simulink model "QRsim"  (R2013b)
settings: Solver=ode45  StartTime=0.0  StopTime=15  RelTol=1e-3
values from neighbouring files (symbols this model uses):
  b = 1    [QRrunfile.m]    (also in develop.m = 0.1)
  d = 8.004e-4    (= 0.0008004)    [QRrunfile.m]    (also in develop.m = 0.1)
  DeltaR = [0; 0; 0]    [QRrunfile.m]
  Deltax = [0; 0; 0]    [QRrunfile.m]
  dphi0 = 0    [QRrunfile.m]    (also in develop.m)
  dpsi0 = 0    [QRrunfile.m]    (also in develop.m)
  dtheta0 = 0    [QRrunfile.m]    (also in develop.m)
  dx0 = 0    [QRrunfile.m]    (also in develop.m)
  dy0 = 0    [QRrunfile.m]    (also in develop.m)
  dz0 = 0    [QRrunfile.m]    (also in develop.m)
  e3 = [0;0;1]    [QRrunfile.m]
  g = 9.81    [QRrunfile.m]    (also in develop.m)
  I = diag([Ixx Iyy Izz])    [QRrunfile.m]    (also in develop.m)
  Ir = 0    [QRrunfile.m]    (also in develop.m = 0.5)
  Ixx = 0.0820    (= 0.082)    [QRrunfile.m]    (also in develop.m = 1.5)
  Iyy = 0.0845    [QRrunfile.m]    (also in develop.m = 1.5)
  Izz = .1377    (= 0.1377)    [QRrunfile.m]    (also in develop.m = 1.5)
  kOmega = kOmega_phi*eye(3)    [QRrunfile.m]
  kR = kR_phi*eye(3)    [QRrunfile.m]
  kv = 5.6*m    (= 24.304)    [QRrunfile.m]
  kx = 16*m    (= 69.44)    [QRrunfile.m]
  l = 0.315    [QRrunfile.m]    (also in develop.m = 0.12)
  m = 4.34    [QRrunfile.m]    (also in develop.m = 0.42)
  phi0 = pi/8    (= 0.392699081699)    [QRrunfile.m]    (also in develop.m = 0)
  psi0 = 0    [QRrunfile.m]    (also in develop.m)
  theta0 = 0    [QRrunfile.m]    (also in develop.m)
  x0 = 0    [QRrunfile.m]    (also in develop.m)
  y0 = 0    [QRrunfile.m]    (also in develop.m)
  z0 = 0    [QRrunfile.m]    (also in develop.m)
undefined symbols (not defined in the file or in its folder): sigbuilder_block
libraries: dspsrcs4 x3, simulink_extras x3, vrlib x1
settings Model: Creator=Nam  LastModifiedBy=Nam
settings DataIOCC: SaveFormat=StructureWithTime
settings DebuggingCC: SolverPrmCheckMsg=none

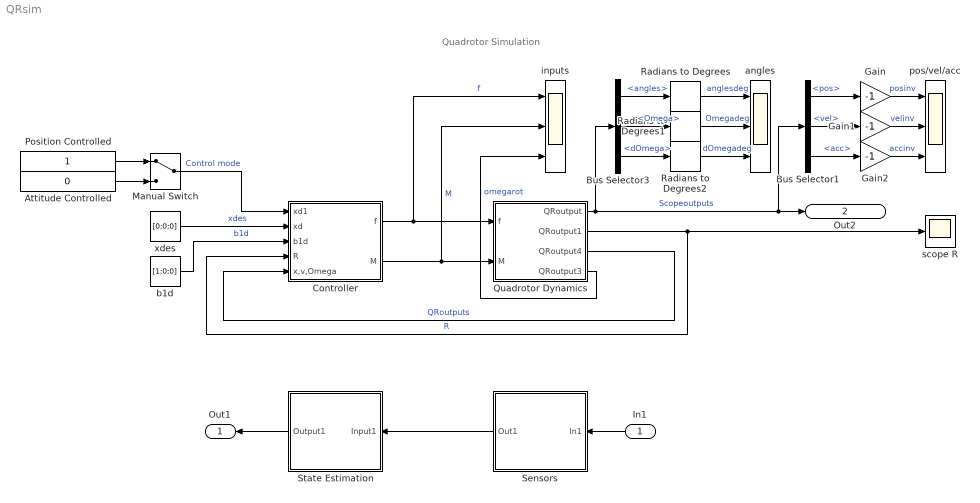
== system QRsim ==
  note: Quadrotor Simulation
  In1 : Inport
  Attitude Controlled : Constant  Value=0  VectorParams1D=off
      mask Display: disp('Attitude controlled')
  Bus Selector1 : BusSelector  OutputSignals=signal1.pos,signal1.vel,signal1.acc
  Bus Selector3 : BusSelector  OutputSignals=signal2.angles,signal2.Omega,signal2.dOmega
  Controller : Subsystem
      mask Display: disp('Controller')
  Gain : Gain  Gain=-1
  Gain1 : Gain  Gain=-1
  Gain2 : Gain  Gain=-1
  Manual Switch : ManualSwitch
  Position Controlled : Constant  VectorParams1D=off
      mask Display: disp('Position controlled')
  Quadrotor Dynamics : Subsystem
      mask Display: image('bebop.png')
  Radians to Degrees : simulink_extras/Transformations/Radians to Degrees
  Radians to Degrees1 : simulink_extras/Transformations/Radians to Degrees
  Radians to Degrees2 : simulink_extras/Transformations/Radians to Degrees
  Sensors : Subsystem
      mask Display: image('optitrack.jpg')
  State Estimation : Subsystem
  angles : Scope  NumInputPorts=3
      settings: ShowLegends=on  YMin=-375~-850~-1e+13  YMax=25~0~1e+12
  b1d : Constant  Value=[1;0;0]  VectorParams1D=off
  inputs : Scope  NumInputPorts=3
      settings: ShowLegends=on  YMin=-5~-5~-5  YMax=5~5~5  SaveName=ScopeData2
  pos/vel/acc : Scope  NumInputPorts=3
      settings: ShowLegends=on  YMin=-5~-5~-5  YMax=5~5~5
  scope R : Scope
      settings: SaveName=ScopeData16
  xdes : Constant  Value=[0;0;0]  VectorParams1D=off
  Out1 : Outport
  Out2 : Outport  Port=2
  wires:
  Sensors/1(Out1) -> State Estimation/1(Input1)
  xdes/1 -> Controller/2(xd)  "xdes"
  b1d/1 -> Controller/3(b1d)  "b1d"
  State Estimation/1(Output1) -> Out1/1
  In1/1 -> Sensors/1(In1)
  Controller/1(f) -> Quadrotor Dynamics/1(f), inputs/1  "f"
  Controller/2(M) -> Quadrotor Dynamics/2(M), inputs/2  "M"
  Quadrotor Dynamics/1(QRoutput) -> Bus Selector1/1, Out2/1, Bus Selector3/1  "Scopeoutputs"
  Bus Selector3/1 -> Radians to Degrees/1  "<angles>"
  Bus Selector3/2 -> Radians to Degrees1/1  "<Omega>"
  Bus Selector3/3 -> Radians to Degrees2/1  "<dOmega>"
  Gain/1 -> pos/vel/acc/1  "posinv"
  Gain1/1 -> pos/vel/acc/2  "velinv"
  Gain2/1 -> pos/vel/acc/3  "accinv"
  Bus Selector1/1 -> Gain/1  "<pos>"
  Bus Selector1/2 -> Gain1/1  "<vel>"
  Bus Selector1/3 -> Gain2/1  "<acc>"
  Quadrotor Dynamics/4(QRoutput3) -> inputs/3  "omegarot"
  Quadrotor Dynamics/2(QRoutput1) -> scope R/1, Controller/4(R)  "R"
  Quadrotor Dynamics/3(QRoutput4) -> Controller/5(x,v,Omega)  "QRoutputs"
  Radians to Degrees/1 -> angles/1  "anglesdeg"
  Radians to Degrees1/1 -> angles/2  "Omegadeg"
  Radians to Degrees2/1 -> angles/3  "dOmegadeg"
  Position Controlled/1 -> Manual Switch/1
  Attitude Controlled/1 -> Manual Switch/2
  Manual Switch/1 -> Controller/1(xd1)  "Control mode"

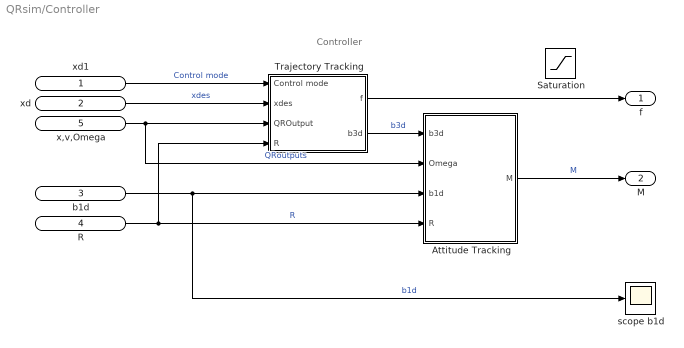
== system QRsim/Controller ==
  note: Controller
  xd1 : Inport
  xd : Inport  Port=2
  b1d : Inport  Port=3
  R : Inport  Port=4
  x,v,Omega : Inport  Port=5
  Attitude Tracking : Subsystem
      mask Display: disp('Attitude\nTracking')
  Saturation : Saturate  UpperLimit=200  LowerLimit=-200
  Trajectory Tracking : Subsystem
      mask Display: disp('Trajectory\nTracking')
  scope b1d : Scope
      settings: SaveName=ScopeData5
  f : Outport
  M : Outport  Port=2
  wires:
  b1d/1 -> scope b1d/1, Attitude Tracking/3(b1d)  "b1d"
  Attitude Tracking/1(M) -> M/1  "M"
  xd/1 -> Trajectory Tracking/2(xdes)  "xdes"
  Trajectory Tracking/2(b3d) -> Attitude Tracking/1(b3d)  "b3d"
  R/1 -> Trajectory Tracking/4(R), Attitude Tracking/4(R)  "R"
  x,v,Omega/1 -> Attitude Tracking/2(Omega), Trajectory Tracking/3(QROutput)  "QRoutputs"
  Trajectory Tracking/1(f) -> f/1
  xd1/1 -> Trajectory Tracking/1(Control mode)  "Control mode"

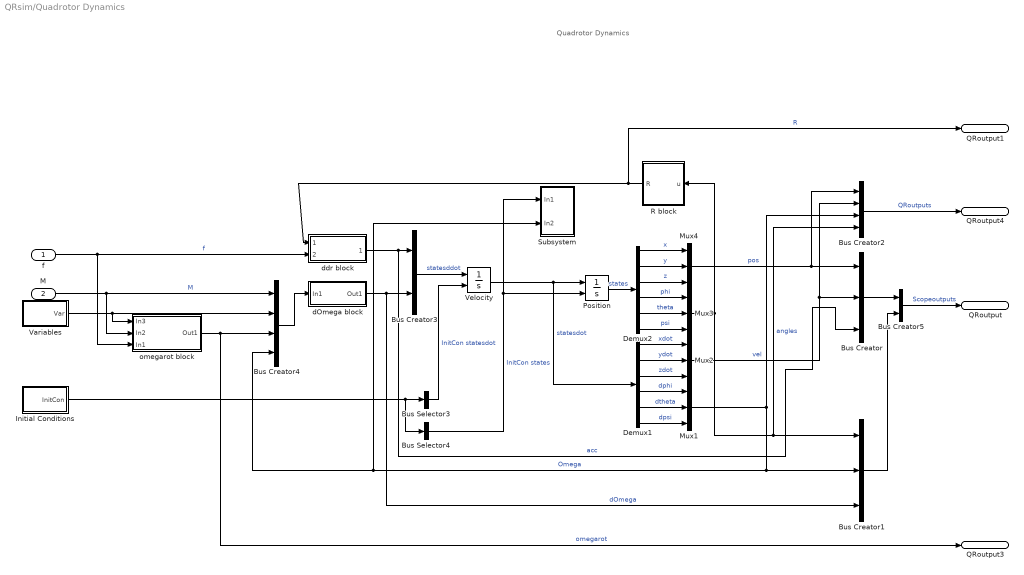
== system QRsim/Quadrotor Dynamics ==
  note: Quadrotor Dynamics
  f : Inport
  M : Inport  Port=2  PortDimensions=[3 1]
  Bus Creator : BusCreator  Inputs=3
  Bus Creator1 : BusCreator  Inputs=3
  Bus Creator2 : BusCreator
  Bus Creator3 : BusCreator  Inputs=2
  Bus Creator4 : BusCreator
  Bus Creator5 : BusCreator  Inputs=2
  Bus Selector3 : BusSelector  OutputSignals=InitCon dot.dx0,InitCon dot.dy0,InitCon dot.dz0,InitCon dot.dphi0,InitCon dot.dtheta0,InitCon dot.dpsi0  OutputAsBus=on
  Bus Selector4 : BusSelector  OutputSignals=InitCon.x0,InitCon.y0,InitCon.z0,InitCon.phi0,InitCon.theta0,InitCon.psi0  OutputAsBus=on
  Demux1 : Demux  Outputs=6
  Demux2 : Demux  Outputs=6
  Initial Conditions : Subsystem
  Mux{1..4} (4 alike) : Mux  Inputs=3
  Position : Integrator  InitialConditionSource=external
  R block : MATLAB Function  TreatAsAtomicUnit=on
  Subsystem : Subsystem
  Variables : Subsystem
      mask Display: disp('Variables')
  Velocity : Integrator  InitialConditionSource=external
  dOmega block : Subsystem
      mask Display: disp('[\psi{"}; \phi{"}; \theta{"}]','texmode','on')
  ddr block : Subsystem
      mask Display: disp('[x{"}; y{"}; z{"}]','texmode','on')
  omegarot block : Subsystem
      mask Display: disp('(f,M) \rightarrow \omega_i','texmode','on')
  QRoutput : Outport
  QRoutput1 : Outport  Port=2
  QRoutput4 : Outport  Port=3
  QRoutput3 : Outport  Port=4
  wires:
  Velocity/1 -> Position/1, Demux1/1  "statesdot"
  f/1 -> ddr block/2(R,f,m,g), omegarot block/3(In1)  "f"
  Variables/1(Var) -> omegarot block/1(In3), Bus Creator4/2
  M/1 -> omegarot block/2(In2), Bus Creator4/1  "M"
  Position/1 -> Demux2/1  "states"
  ddr block/1(rddotOutput) -> Bus Creator/3, Bus Creator3/1  "acc"
  Bus Creator3/1 -> Velocity/1  "statesddot"
  Initial Conditions/1(InitCon) -> Bus Selector3/1, Bus Selector4/1
  Bus Selector3/1 -> Velocity/2  "InitCon statesdot"
  Bus Selector4/1 -> Subsystem/1(In1), Position/2  "InitCon states"
  dOmega block/1(Out1) -> Bus Creator3/2, Bus Creator1/3  "dOmega"
  Bus Creator4/1 -> dOmega block/1(In1)
  Demux1/4 -> Mux1/1  "dphi"
  Demux1/5 -> Mux1/2  "dtheta"
  Demux1/6 -> Mux1/3  "dpsi"
  Demux1/2 -> Mux2/2  "ydot"
  Demux1/1 -> Mux2/1  "xdot"
  Demux1/3 -> Mux2/3  "zdot"
  Mux2/1 -> Bus Creator2/2, Bus Creator/2  "vel"
  Demux2/4 -> Mux3/1  "phi"
  Demux2/5 -> Mux3/2  "theta"
  Demux2/6 -> Mux3/3  "psi"
  Demux2/2 -> Mux4/2  "y"
  Demux2/1 -> Mux4/1  "x"
  Demux2/3 -> Mux4/3  "z"
  Mux3/1 -> Bus Creator2/4, Bus Creator1/1, R block/1(u)  "angles"
  Mux4/1 -> Bus Creator2/1, Bus Creator/1  "pos"
  omegarot block/1(Out1) -> QRoutput3/1, Bus Creator4/3  "omegarot"
  Bus Creator/1 -> Bus Creator5/1
  Bus Creator1/1 -> Bus Creator5/2
  Bus Creator5/1 -> QRoutput/1  "Scopeoutputs"
  Mux1/1 -> Subsystem/2(In2), Bus Creator4/4, Bus Creator1/2, Bus Creator2/3  "Omega"
  Bus Creator2/1 -> QRoutput4/1  "QRoutputs"
  R block/1(R) -> QRoutput1/1, ddr block/1(R,f,m,g1)  "R"

== system QRsim/Sensors ==
  In1 : Inport
  Out1 : Outport
  wires:
  In1/1 -> Out1/1

== system QRsim/State Estimation ==
  Input1 : Inport
  Output1 : Outport
  wires:
  Input1/1 -> Output1/1

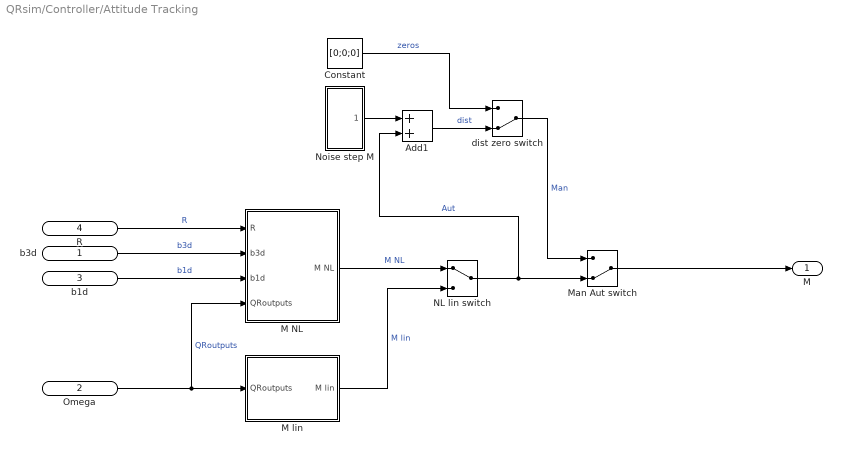
== system QRsim/Controller/Attitude Tracking ==
  b3d : Inport
  Omega : Inport  Port=2
  b1d : Inport  Port=3
  R : Inport  Port=4
  Add1 : Sum
  Constant : Constant  Value=[0;0;0]
  M NL : Subsystem
  M lin : Subsystem
  Man Aut switch : ManualSwitch  CurrentSetting=0
  NL lin switch : ManualSwitch
  Noise step M : Subsystem
  dist zero switch : ManualSwitch  CurrentSetting=0
  M : Outport
  wires:
  M NL/1(M NL) -> NL lin switch/1  "M NL"
  R/1 -> M NL/1(R)  "R"
  b3d/1 -> M NL/2(b3d)  "b3d"
  b1d/1 -> M NL/3(b1d)  "b1d"
  Omega/1 -> M NL/4(QRoutputs), M lin/1(QRoutputs)  "QRoutputs"
  M lin/1(M lin) -> NL lin switch/2  "M lin"
  Noise step M/1(Out1) -> Add1/1
  Constant/1 -> dist zero switch/1  "zeros"
  Add1/1 -> dist zero switch/2  "dist"
  dist zero switch/1 -> Man Aut switch/1  "Man"
  NL lin switch/1 -> Add1/2, Man Aut switch/2  "Aut"
  Man Aut switch/1 -> M/1

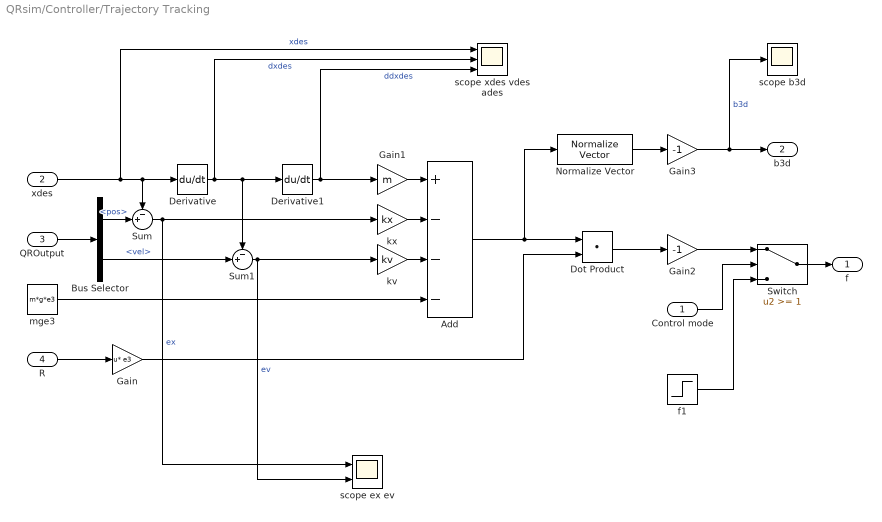
== system QRsim/Controller/Trajectory Tracking ==
  Control mode : Inport
  xdes : Inport  Port=2
  QROutput : Inport  Port=3
  R : Inport  Port=4
  Add : Sum  Inputs=+---
  Bus Selector : BusSelector  OutputSignals=pos,vel
  Derivative : Derivative
  Derivative1 : Derivative
  Dot Product : DotProduct  InputSameDT=on  OutDataTypeStr=Inherit: Inherit via internal rule
  Gain : Gain  Gain=e3  Multiplication=Matrix(u*K)
  Gain1 : Gain  Gain=m
  Gain2 : Gain  Gain=-1
  Gain3 : Gain  Gain=-1
  Normalize Vector : vrlib/Utilities/Normalize Vector  maxzero=0
  Sum : Sum  Inputs=-+|
  Sum1 : Sum  Inputs=-+|
  Switch : Switch  Threshold=1
  f1 : Step  Time=0  After=m*g  SampleTime=0
  kv : Gain  Gain=kv
  kx : Gain  Gain=kx
  mge3 : Constant  Value=m*g*e3  VectorParams1D=off
  scope b3d : Scope
      settings: SaveName=ScopeData4
  scope ex ev : Scope  NumInputPorts=2
      settings: YMin=-5~-5  YMax=5~5  SaveName=ScopeData7
  scope xdes vdes ades : Scope  NumInputPorts=3
      settings: YMin=-5~-5~-5  YMax=5~5~5  SaveName=ScopeData6
  f : Outport
  b3d : Outport  Port=2
  wires:
  xdes/1 -> Derivative/1, Sum/1, scope xdes vdes ades/1  "xdes"
  Derivative/1 -> Derivative1/1, Sum1/1, scope xdes vdes ades/2  "dxdes"
  Derivative1/1 -> Gain1/1, scope xdes vdes ades/3  "ddxdes"
  QROutput/1 -> Bus Selector/1
  Bus Selector/1 -> Sum/2  "<pos>"
  Bus Selector/2 -> Sum1/2  "<vel>"
  R/1 -> Gain/1
  Sum1/1 -> scope ex ev/2, kv/1  "ev"
  Sum/1 -> scope ex ev/1, kx/1  "ex"
  Gain1/1 -> Add/1
  kx/1 -> Add/2
  kv/1 -> Add/3
  mge3/1 -> Add/4
  Dot Product/1 -> Gain2/1
  Add/1 -> Normalize Vector/1, Dot Product/1
  Gain/1 -> Dot Product/2
  Normalize Vector/1 -> Gain3/1
  Gain3/1 -> scope b3d/1, b3d/1  "b3d"
  Gain2/1 -> Switch/1
  f1/1 -> Switch/3
  Switch/1 -> f/1
  Control mode/1 -> Switch/2

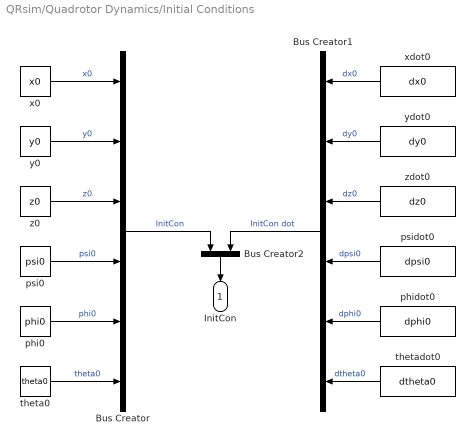
== system QRsim/Quadrotor Dynamics/Initial Conditions ==
  Bus Creator : BusCreator  Inputs=6
  Bus Creator1 : BusCreator  Inputs=6
  Bus Creator2 : BusCreator  Inputs=2
  phi0 : Constant  Value=phi0
  phidot0 : Constant  Value=dphi0
  psi0 : Constant  Value=psi0
  psidot0 : Constant  Value=dpsi0
  theta0 : Constant  Value=theta0
  thetadot0 : Constant  Value=dtheta0
  x0 : Constant  Value=x0
  xdot0 : Constant  Value=dx0
  y0 : Constant  Value=y0
  ydot0 : Constant  Value=dy0
  z0 : Constant  Value=z0
  zdot0 : Constant  Value=dz0
  InitCon : Outport
  wires:
  phi0/1 -> Bus Creator/5  "phi0"
  y0/1 -> Bus Creator/2  "y0"
  psi0/1 -> Bus Creator/4  "psi0"
  x0/1 -> Bus Creator/1  "x0"
  z0/1 -> Bus Creator/3  "z0"
  theta0/1 -> Bus Creator/6  "theta0"
  Bus Creator1/1 -> Bus Creator2/2  "InitCon dot"
  psidot0/1 -> Bus Creator1/4  "dpsi0"
  xdot0/1 -> Bus Creator1/1  "dx0"
  zdot0/1 -> Bus Creator1/3  "dz0"
  ydot0/1 -> Bus Creator1/2  "dy0"
  phidot0/1 -> Bus Creator1/5  "dphi0"
  thetadot0/1 -> Bus Creator1/6  "dtheta0"
  Bus Creator2/1 -> InitCon/1
  Bus Creator/1 -> Bus Creator2/1  "InitCon"

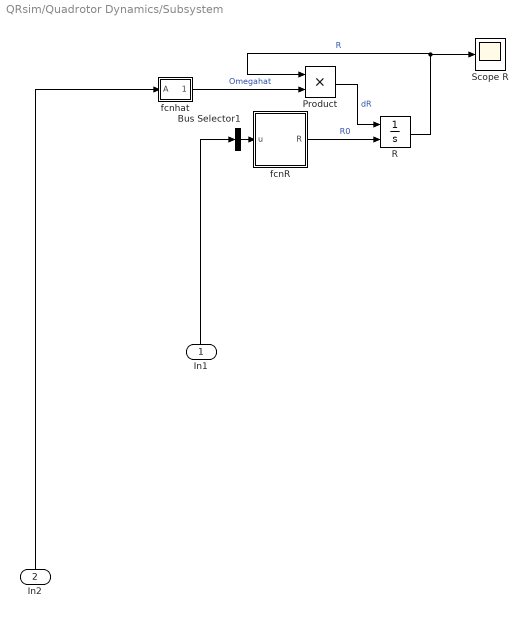
== system QRsim/Quadrotor Dynamics/Subsystem ==
  In1 : Inport
  In2 : Inport  Port=2
  Bus Selector1 : BusSelector  OutputSignals=phi0,theta0,psi0  OutputAsBus=on
  Product : Product
  R : Integrator  InitialConditionSource=external
  Scope R : Scope
      settings: ShowLegends=on  SaveName=ScopeData9
  fcnR : MATLAB Function  TreatAsAtomicUnit=on
  fcnhat : MATLAB Function  TreatAsAtomicUnit=on
  wires:
  Bus Selector1/1 -> fcnR/1(u)
  In2/1 -> fcnhat/1(A)
  In1/1 -> Bus Selector1/1
  fcnhat/1(fcnhat) -> Product/2  "Omegahat"
  fcnR/1(R) -> R/2  "R0"
  Product/1 -> R/1  "dR"
  R/1 -> Scope R/1, Product/1  "R"

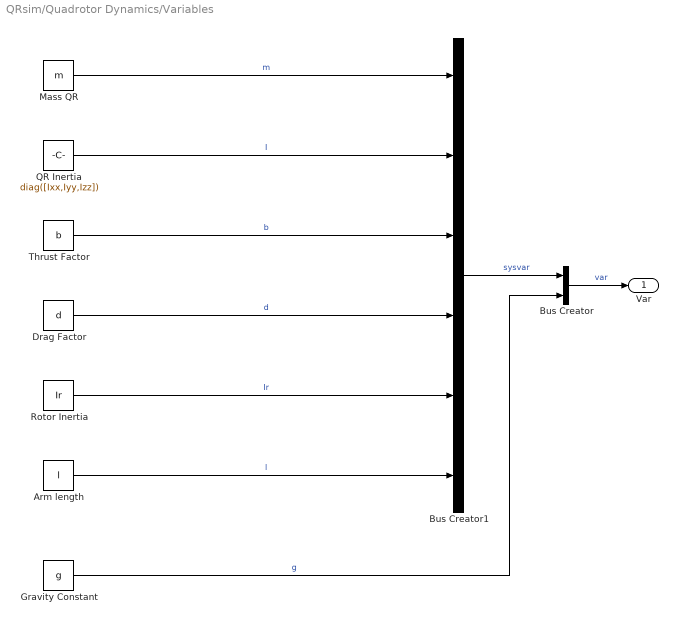
== system QRsim/Quadrotor Dynamics/Variables ==
  Arm length : Constant  Value=l
  Bus Creator : BusCreator  Inputs=2
  Bus Creator1 : BusCreator  Inputs=6
  Drag Factor : Constant  Value=d
  Gravity Constant : Constant  Value=g
  Mass QR : Constant  Value=m
  QR Inertia : Constant  Value=diag([Ixx,Iyy,Izz])
  Rotor Inertia : Constant  Value=Ir
  Thrust Factor : Constant  Value=b
  Var : Outport
  wires:
  Gravity Constant/1 -> Bus Creator/2  "g"
  Bus Creator/1 -> Var/1  "var"
  Mass QR/1 -> Bus Creator1/1  "m"
  Arm length/1 -> Bus Creator1/6  "l"
  Rotor Inertia/1 -> Bus Creator1/5  "Ir"
  QR Inertia/1 -> Bus Creator1/2  "I"
  Bus Creator1/1 -> Bus Creator/1  "sysvar"
  Thrust Factor/1 -> Bus Creator1/3  "b"
  Drag Factor/1 -> Bus Creator1/4  "d"

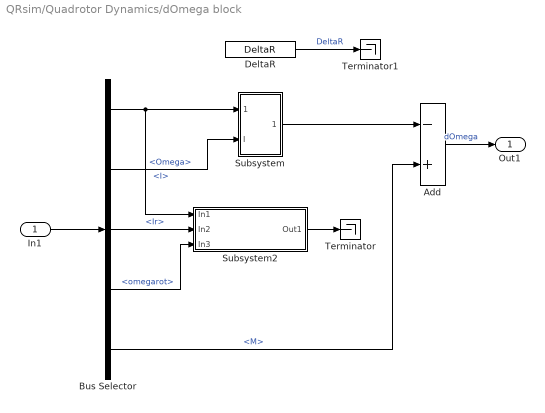
== system QRsim/Quadrotor Dynamics/dOmega block ==
  In1 : Inport
  Add : Sum  Inputs=-+
  Bus Selector : BusSelector  OutputSignals=Omega,var.sysvar.I,var.sysvar.Ir,omegarot,M
  DeltaR : Constant  Value=DeltaR
      mask Display: disp('\Delta_R','texmode','on')
  Subsystem : Subsystem
      mask Display: disp('\Omega \times I\Omega','texmode','on')
  Subsystem2 : Subsystem
      mask Display: disp('\tau_G=\Sigma I_R(\omega \times e_3) \omega_i ','texmode','on')
  Terminator : Terminator
  Terminator1 : Terminator
  Out1 : Outport
  wires:
  In1/1 -> Bus Selector/1
  Add/1 -> Out1/1  "dOmega"
  Bus Selector/1 -> Subsystem/1(Omega), Subsystem2/1(In1)  "<Omega>"
  Bus Selector/2 -> Subsystem/2(I)  "<I>"
  Subsystem/1(Out1) -> Add/1
  Bus Selector/3 -> Subsystem2/2(In2)  "<Ir>"
  Bus Selector/5 -> Add/2  "<M>"
  Subsystem2/1(Out1) -> Terminator/1
  Bus Selector/4 -> Subsystem2/3(In3)  "<omegarot>"
  DeltaR/1 -> Terminator1/1  "DeltaR"

== system QRsim/Quadrotor Dynamics/ddr block ==
  R,f,m,g1 : Inport
  R,f,m,g : Inport  Port=2
  Deltax : Constant  Value=Deltax
      mask Display: disp('\Delta_x','texmode','on')
  fcnddr : MATLAB Function  TreatAsAtomicUnit=on
  g : Constant  Value=g
  m : Constant  Value=m
  rddotOutput : Outport
  wires:
  fcnddr/1(ddr) -> rddotOutput/1  "ddr"
  R,f,m,g/1 -> fcnddr/2(f)  "f"
  R,f,m,g1/1 -> fcnddr/1(R)  "R"
  m/1 -> fcnddr/3(m)  "m"
  g/1 -> fcnddr/4(g)  "g"
  Deltax/1 -> fcnddr/5(Deltax)  "Deltax"

== system QRsim/Quadrotor Dynamics/omegarot block ==
  In3 : Inport
  In2 : Inport  Port=2
  In1 : Inport  Port=3
  Bus Selector2 : BusSelector  OutputSignals=sysvar.b,sysvar.d,sysvar.l  OutputAsBus=on
  Saturation : Saturate  UpperLimit=inf  LowerLimit=0
  Sqrt : Sqrt  SaturateOnIntegerOverflow=on
  fcnomega : MATLAB Function  TreatAsAtomicUnit=on
  Out1 : Outport
  wires:
  In3/1 -> Bus Selector2/1
  In1/1 -> fcnomega/2(f)  "f"
  In2/1 -> fcnomega/3(M)  "M"
  Bus Selector2/1 -> fcnomega/1(var)  "var"
  Sqrt/1 -> Out1/1  "omega"
  Saturation/1 -> Sqrt/1
  fcnomega/1(omega) -> Saturation/1  "omega"

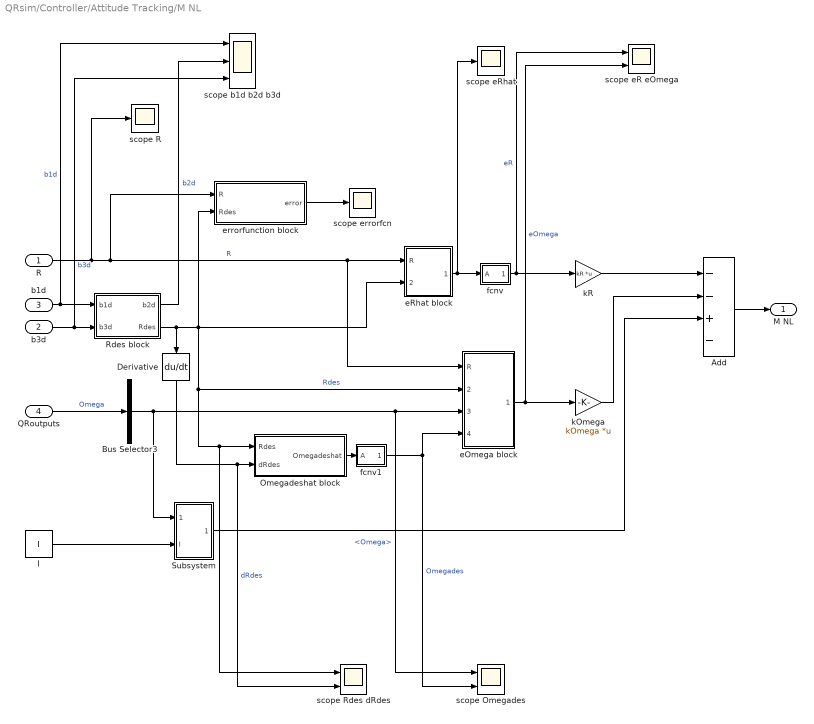
== system QRsim/Controller/Attitude Tracking/M NL ==
  R : Inport
  b3d : Inport  Port=2
  b1d : Inport  Port=3
  QRoutputs : Inport  Port=4
  Add : Sum  Inputs=--+-
  Bus Selector3 : BusSelector  OutputSignals=Omega
  Derivative : Derivative
  I : Constant  Value=I
  Omegadeshat block : MATLAB Function  TreatAsAtomicUnit=on
  Rdes block : MATLAB Function  TreatAsAtomicUnit=on
  Subsystem : Subsystem
      mask Display: disp('\Omega \times I\Omega','texmode','on')
  eOmega block : MATLAB Function  TreatAsAtomicUnit=on
  eRhat block : MATLAB Function  TreatAsAtomicUnit=on
  errorfunction block : MATLAB Function  TreatAsAtomicUnit=on
  fcnv : MATLAB Function  TreatAsAtomicUnit=on
  fcnv1 : MATLAB Function  TreatAsAtomicUnit=on
  kOmega : Gain  Gain=kOmega  Multiplication=Matrix(K*u)
  kR : Gain  Gain=kR  Multiplication=Matrix(K*u)
  scope Omegades : Scope  NumInputPorts=2
      settings: ShowLegends=on  YMin=-5~-5  YMax=5~5  SaveName=ScopeData12
  scope R : Scope
      settings: SaveName=ScopeData14
  scope Rdes dRdes : Scope  NumInputPorts=2
      settings: YMin=-5~-5  YMax=5~5  SaveName=ScopeData11
  scope b1d b2d b3d : Scope  NumInputPorts=3
      settings: ShowLegends=on  YMin=-5~-5~-5  YMax=5~5~5  SaveName=ScopeData10
  scope eR eOmega : Scope  NumInputPorts=2
      settings: YMin=-5~-5  YMax=5~5  SaveName=ScopeData8
  scope eRhat : Scope
      settings: SaveName=ScopeData13
  scope errorfcn : Scope
      settings: SaveName=ScopeData15
  M NL : Outport
  wires:
  R/1 -> eOmega block/1(R), eRhat block/1(R), errorfunction block/1(R), scope R/1  "R"
  eRhat block/1(eRhat) -> scope eRhat/1, fcnv/1(A)
  fcnv/1(fcnv) -> scope eR eOmega/1, kR/1  "eR"
  kR/1 -> Add/1
  kOmega/1 -> Add/2
  eOmega block/1(eOmega) -> scope eR eOmega/2, kOmega/1  "eOmega"
  b3d/1 -> scope b1d b2d b3d/3, Rdes block/2(b3d)  "b3d"
  b1d/1 -> scope b1d b2d b3d/1, Rdes block/1(b1d)  "b1d"
  QRoutputs/1 -> Bus Selector3/1  "Omega"
  Bus Selector3/1 -> Subsystem/1(Omega), eOmega block/3(Omega), scope Omegades/1  "<Omega>"
  Rdes block/2(Rdes) -> Derivative/1, scope Rdes dRdes/1, Omegadeshat block/1(Rdes), eOmega block/2(Rdes), errorfunction block/2(Rdes), eRhat block/2(Rdes)  "Rdes"
  Omegadeshat block/1(Omegadeshat) -> fcnv1/1(A)
  Derivative/1 -> scope Rdes dRdes/2, Omegadeshat block/2(dRdes)  "dRdes"
  fcnv1/1(fcnv) -> scope Omegades/2, eOmega block/4(Omegades)  "Omegades"
  Rdes block/1(b2d) -> scope b1d b2d b3d/2  "b2d"
  I/1 -> Subsystem/2(I)
  Subsystem/1(Out1) -> Add/3
  Add/1 -> M NL/1
  errorfunction block/1(error) -> scope errorfcn/1

== system QRsim/Controller/Attitude Tracking/M lin ==
  QRoutputs : Inport
  Add : Sum  Inputs=--
  Bus Selector3 : BusSelector  OutputSignals=angles,Omega
  Constant : Constant  Value=[0;0;0]
  eR lin block : MATLAB Function  TreatAsAtomicUnit=on
  kOmega : Gain  Gain=kOmega  Multiplication=Matrix(K*u)
  kR : Gain  Gain=kR  Multiplication=Matrix(K*u)
  M lin : Outport
  wires:
  QRoutputs/1 -> Bus Selector3/1
  Bus Selector3/1 -> eR lin block/2(angles)  "<angles>"
  Bus Selector3/2 -> kOmega/1  "<Omega>"
  eR lin block/1(eRlin) -> kR/1  "eR lin"
  kR/1 -> Add/1
  kOmega/1 -> Add/2
  Add/1 -> M lin/1  "M lin"
  Constant/1 -> eR lin block/1(anglesdes)  "anglesdes"

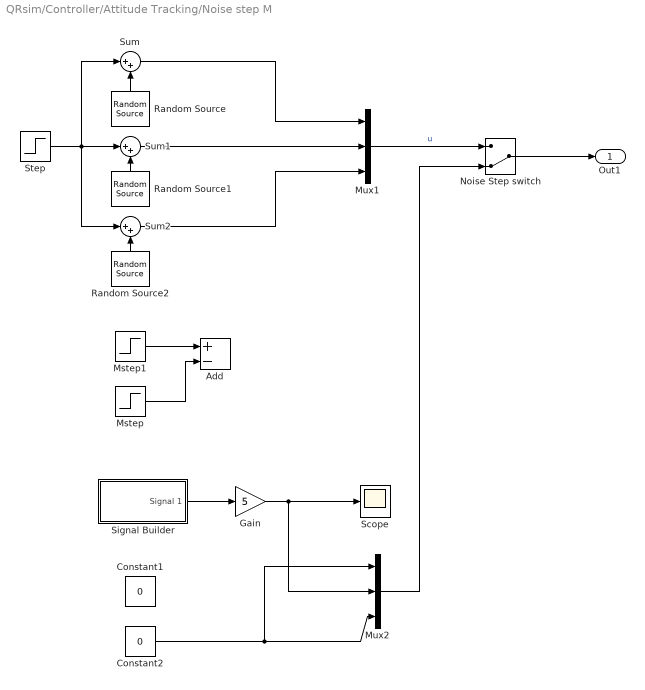
== system QRsim/Controller/Attitude Tracking/Noise step M ==
  Add : Sum  Inputs=+-
  Constant1 : Constant  Value=0
  Constant2 : Constant  Value=0
  Gain : Gain  Gain=5
  Mstep : Step  Time=6  SampleTime=0
  Mstep1 : Step  Time=5  SampleTime=0
  Mux1 : Mux  Inputs=3
  Mux2 : Mux  Inputs=3
  Noise Step switch : ManualSwitch  CurrentSetting=0
  Random Source : dspsrcs4/Random Source  SrcType=Uniform  NormMethod=Ziggurat  CltLength=12  MinVal=0  MaxVal=.1  MeanVal=0  VarVal=1  RepMode=Not repeatable  rawSeed=1  IsInherit=off  SampMode=Continuous  SampTime=1  SampFrame=1  DataType=Double  OutComplex=Real
  Random Source1 : dspsrcs4/Random Source  SrcType=Uniform  NormMethod=Ziggurat  CltLength=12  MinVal=0  MaxVal=.1  MeanVal=0  VarVal=1  RepMode=Not repeatable  rawSeed=1  IsInherit=off  SampMode=Continuous  SampTime=1  SampFrame=1  DataType=Double  OutComplex=Real
  Random Source2 : dspsrcs4/Random Source  SrcType=Uniform  NormMethod=Ziggurat  CltLength=12  MinVal=0  MaxVal=.1  MeanVal=0  VarVal=1  RepMode=Not repeatable  rawSeed=1  IsInherit=off  SampMode=Continuous  SampTime=1  SampFrame=1  DataType=Double  OutComplex=Real
  Scope : Scope
      settings: SaveName=ScopeData3
  Signal Builder : Subsystem  Tag=STV Subsys  LoadFcn=sigbuilder_block('load');  StartFcn=sigbuilder_block('start');  StopFcn=sigbuilder_block('stop');  ClipboardFcn=sigbuilder_block('clipboard');  mask(Sigbuilder block){}
      mask help: Simulink:masks:SigbuilderBlock_MD
      mask init:
      | if ~strcmp(get_param(bdroot(gcbh),'SimulationStatus'),'stopped') tuvar = sigbuilder_block('maskInit'); end
      settings: CopyFcn=sigbuilder_block('copy');  DeleteFcn=sigbuilder_block('delete');  ModelCloseFcn=sigbuilder_block('modelClose');  PreSaveFcn=sigbuilder_block('preSave');  PauseFcn=sigbuilder_block('pause');  ContinueFcn=sigbuilder_block('continue');  NameChangeFcn=sigbuilder_block('namechange');  OpenFcn=sigbuilder_block('open',[437.25 199.5 715.5 399.75 ]);  CloseFcn=sigbuilder_block('close');
      mask Display: plot(0, 0, 100, 100,[2, 2, 32, 32, 2], [68, 8, 8, 68, 68],[32, 2], [38, 38], [32, 19, 2],[53, 60, 44], [32, 17, 17, 2],[16, 16, 31, 31]);txt = getActiveGroup(gcbh);text(2, 100, txt,'verticalAlignment', 'top');
  Step : Step  Time=0  After=0  SampleTime=0
  Sum : Sum  Inputs=|++
  Sum1 : Sum  Inputs=|++
  Sum2 : Sum  Inputs=|++
  Out1 : Outport
  wires:
  Sum/1 -> Mux1/1
  Sum2/1 -> Mux1/3
  Sum1/1 -> Mux1/2
  Random Source1/1 -> Sum1/2
  Mux1/1 -> Noise Step switch/1  "u"
  Random Source/1 -> Sum/2
  Random Source2/1 -> Sum2/2
  Step/1 -> Sum2/1, Sum1/1, Sum/1
  Constant2/1 -> Mux2/1, Mux2/3
  Mux2/1 -> Noise Step switch/2
  Noise Step switch/1 -> Out1/1
  Mstep1/1 -> Add/1
  Mstep/1 -> Add/2
  Signal Builder/1(Signal 1) -> Gain/1
  Gain/1 -> Mux2/2, Scope/1

== system QRsim/Quadrotor Dynamics/dOmega block/Subsystem ==
  Omega : Inport
  I : Inport  Port=2
  Product : Product  Inputs=3  Multiplication=Matrix(*)
  fcnhat : MATLAB Function  TreatAsAtomicUnit=on
  Out1 : Outport
  wires:
  Omega/1 -> Product/3, fcnhat/1(A)
  fcnhat/1(fcnhat) -> Product/1
  I/1 -> Product/2
  Product/1 -> Out1/1

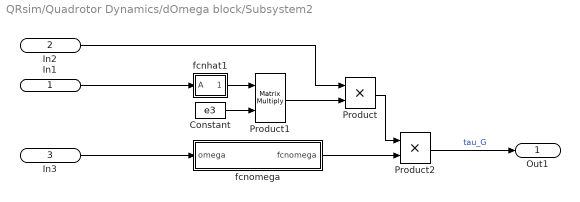
== system QRsim/Quadrotor Dynamics/dOmega block/Subsystem2 ==
  In1 : Inport
  In2 : Inport  Port=2
  In3 : Inport  Port=3
  Constant : Constant  Value=e3
  Product : Product
  Product1 : Product  Multiplication=Matrix(*)
  Product2 : Product
  fcnhat1 : MATLAB Function  TreatAsAtomicUnit=on
  fcnomega : MATLAB Function  TreatAsAtomicUnit=on
  Out1 : Outport
  wires:
  Product2/1 -> Out1/1  "tau_G"
  In2/1 -> Product/1
  fcnomega/1(fcnomega) -> Product2/2
  Product1/1 -> Product/2
  In3/1 -> fcnomega/1(omega)
  In1/1 -> fcnhat1/1(A)
  fcnhat1/1(fcnhat) -> Product1/1
  Constant/1 -> Product1/2
  Product/1 -> Product2/1

== system QRsim/Controller/Attitude Tracking/M NL/Subsystem ==
  Omega : Inport
  I : Inport  Port=2
  Product : Product  Inputs=3  Multiplication=Matrix(*)
  fcnhat : MATLAB Function  TreatAsAtomicUnit=on
  Out1 : Outport
  wires:
  Omega/1 -> Product/3, fcnhat/1(A)
  fcnhat/1(fcnhat) -> Product/1
  I/1 -> Product/2
  Product/1 -> Out1/1

== system QRsim/Controller/Attitude Tracking/Noise step M/Signal Builder ==
  Demux : Demux  Tag=STV Demux  Outputs=1
  FromWs : FromWorkspace  Tag=STV FromWs  VariableName=tuvar  SampleTime=0
      SigBuilderData=|
      | common.afterFinalStr = 'Extrapolate'
      | common.sampleTime = 0
      | dataSet.timeRange = [0 10]
      | dataSet.name = 'Group 1'
      | sbobj.Groups.Name = 'Group 1'
      | sbobj.Groups.Signals.Name = 'Signal 1'
      | sbobj.Groups.Signals.XData = [0 0.5 4.5 5 10]
      | sbobj.Groups.Signals.YData = [0 0.5 0.5 0 0]
  Signal 1 : Outport  Tag=STV Outport
  wires:
  Demux/1 -> Signal 1/1
  FromWs/1 -> Demux/1

== matlab function QRsim/Quadrotor Dynamics/omegarot block/fcnomega ==
  data: var input; f input; M input size=[3 1]; omega output size=[4 1]
function omega = fcn(var,f,M)
%omega = [omega_1^2;omega_2^2;omega_3^2;omega_4^2]

b = var(1);
d = var(2);
l = var(3);

%check if Gamma is invertible?
Gamma = [b b b b;0 -l*b 0 l*b;l*b 0 -l*b 0;-d d -d d];

QRinput = [f;M];

omega = Gamma\QRinput;

== matlab function QRsim/Quadrotor Dynamics/dOmega block/Subsystem/fcnhat ==
  data: A input; fcnhat output
function fcnhat = fcn(A)

a = A(1);
b = A(2);
c = A(3);
fcnhat = [0 -c b; 
          c 0 -a;
         -b a 0];

== matlab function QRsim/Quadrotor Dynamics/ddr block/fcnddr ==
  data: R input size=[3 3]; ddr output size=[3 1]; f input size=1; m input; g input; Deltax input size=[3 1]
function ddr = fcn(R,f,m,g,Deltax)
%ddr = [xddot; yddot; zddot]
%e3 downwards
%m*vdot = g*e_3-f/m*R*e3



ddr = ([0;0;m*g]-f*R*[0;0;1]+Deltax) / m;

== matlab function QRsim/Quadrotor Dynamics/dOmega block/Subsystem2/fcnhat1 ==
  data: A input; fcnhat output
function fcnhat = fcn(A)

a = A(1);
b = A(2);
c = A(3);
fcnhat = [0 -c b; 
          c 0 -a;
         -b a 0];

== matlab function QRsim/Controller/Attitude Tracking/M NL/Omegadeshat block ==
  data: Rdes input size=[3 3]; dRdes input size=[3 3]; Omegadeshat output size=[3 3]
function Omegadeshat = fcn(Rdes,dRdes)
% Rdes = [b1d,b3d x b1d,b3d]

Omegadeshat = Rdes'*dRdes;

== matlab function QRsim/Quadrotor Dynamics/dOmega block/Subsystem2/fcnomega ==
  data: omega input; fcnomega output
function fcnomega = fcn(omega)

fcnomega = omega(2)+omega(4)-omega(1)-omega(3);

== matlab function QRsim/Controller/Attitude Tracking/M NL/Subsystem/fcnhat ==
  data: A input; fcnhat output
function fcnhat = fcn(A)

a = A(1);
b = A(2);
c = A(3);
fcnhat = [0 -c b; 
          c 0 -a;
         -b a 0];

== matlab function QRsim/Controller/Attitude Tracking/M NL/eRhat block ==
  data: R input size=[3 3]; Rdes input size=[3 3]; eRhat output size=[3 3]
function eRhat = fcnR(R,Rdes)
% Z-X-Y psi-phi-theta

eRhat = 0.5*(Rdes'*R-R'*Rdes);

== matlab function QRsim/Controller/Attitude Tracking/M NL/fcnv ==
  data: A input size=[3 3]; fcnv output size=[3 1]
function fcnv = fcn(A)
% Inverse hat function

a    = A(6);
b    = -A(3);
c    = A(2);

fcnv = [a;b;c];

== matlab function QRsim/Controller/Attitude Tracking/M lin/eR lin block ==
  data: anglesdes input size=[3 1]; angles input size=[3 1]; eRlin output size=[3 1]
function eRlin = fcnR(anglesdes,angles)
% Z-X-Y psi-phi-theta
% Rdes =  R(psi0+dpsi, dphi, dtheta)
% R = R(psi0,0,0)

% dphi   = anglesdes(1) - angles(1);
% dtheta = anglesdes(2) - angles(2);
% dpsi   = anglesdes(3) - angles(3);

dphi   = angles(1);
dtheta = angles(2);
dpsi   = angles(3);

eRlin  = [dphi; dtheta; dpsi];
% Of toch: 
% eRlin  = [-dphi; -dtheta; -dpsi];

== matlab function QRsim/Controller/Attitude Tracking/M NL/eOmega block ==
  data: R input size=[3 3]; Rdes input size=[3 3]; eOmega output size=[3 1]; Omega input size=[3 1]; Omegades input size=[3 1]
function eOmega = fcnR(R,Rdes,Omega,Omegades)
% Z-X-Y psi-phi-theta

eOmega = Omega - R'*Rdes*Omegades;

== matlab function QRsim/Controller/Attitude Tracking/M NL/Rdes block ==
  data: b2d output; b1d input size=[3 1]; Rdes output size=[3 3]; b3d input size=[3 1]
function [b2d,Rdes] = fcnRdes(b1d,b3d)
%
b2d = cross(b3d,b1d);
Rdes = [b1d b2d b3d];

== matlab function QRsim/Quadrotor Dynamics/Subsystem/fcnR ==
  data: u input size=[3 1]; R output size=[3 3]
function R = fcnR(u)
% Z-X-Y psi-phi-theta
% u1 = phi, 
% u2 = theta, 
% u3 = psi

phi        = u(1);
theta      = u(2);
psi        = u(3);

R          = [cos(psi)*cos(theta)-sin(phi)*sin(psi)*sin(theta)   -cos(phi)*sin(psi)   cos(psi)*sin(theta)+cos(theta)*sin(phi)*sin(psi);
              cos(theta)*sin(psi)+cos(psi)*sin(phi)*sin(theta)    cos(phi)*cos(psi)   sin(psi)*sin(theta)-cos(psi)*cos(theta)*sin(phi);
             -cos(phi)*sin(theta)                                 sin(phi)            cos(phi)*cos(theta)];

== matlab function QRsim/Controller/Attitude Tracking/M NL/fcnv1 ==
  data: A input size=[3 3]; fcnv output size=[3 1]
function fcnv = fcn(A)
% Inverse hat function

a    = A(6);
b    = -A(3);
c    = A(2);

fcnv = [a;b;c];

== matlab function QRsim/Quadrotor Dynamics/Subsystem/fcnhat ==
  data: A input; fcnhat output
function fcnhat = fcn(A)

a = A(1);
b = A(2);
c = A(3);
fcnhat = [0 -c b; 
          c 0 -a;
         -b a 0];

== matlab function QRsim/Quadrotor Dynamics/R block ==
  data: u input size=[3 1]; R output size=[3 3]
function R = fcnR(u)
% Z-X-Y psi-phi-theta
% u1 = phi, 
% u2 = theta, 
% u3 = psi

phi        = u(1);
theta      = u(2);
psi        = u(3);

R          = [cos(psi)*cos(theta)-sin(phi)*sin(psi)*sin(theta)   -cos(phi)*sin(psi)   cos(psi)*sin(theta)+cos(theta)*sin(phi)*sin(psi);
              cos(theta)*sin(psi)+cos(psi)*sin(phi)*sin(theta)    cos(phi)*cos(psi)   sin(psi)*sin(theta)-cos(psi)*cos(theta)*sin(phi);
             -cos(phi)*sin(theta)                                 sin(phi)            cos(phi)*cos(theta)];

== matlab function QRsim/Controller/Attitude Tracking/M NL/errorfunction block ==
  data: R input size=[3 3]; Rdes input size=[3 3]; error output
function error = fcn(R,Rdes)

error = 0.5*trace(eye(3)-Rdes'*R);
